simulink library "ESTS_UOD_FacOverSteer"  (R2022a)
settings: Solver=VariableStepAuto  StartTime=0.0  StopTime=10.0  RelTol=1e-3
undefined symbols (not defined in the file): ESTS_UOD_c_TiSample_s, ESTS_UOD_p_AgrVSideSlipReDifLatRefLimOS_degps, ESTS_UOD_p_TiTrans_s, ESTS_UOD_p_YawRateDifLatRefLimOS_degps
libraries: VUT_lib x3, simulink x1
settings Model: Creator=blatak  LastModifiedBy=blatak

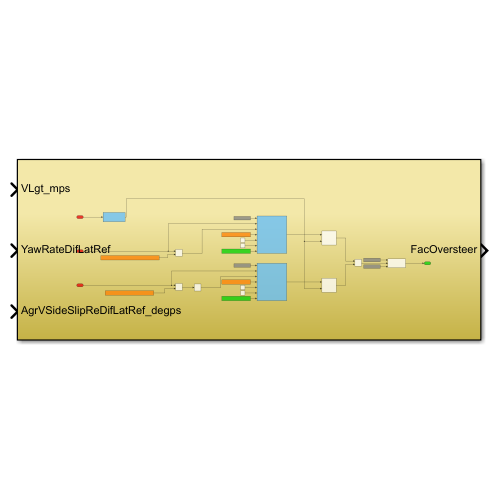
[thumbnail: Simulink's stored preview of the top-level diagram]
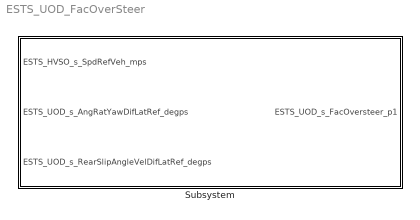
== system ESTS_UOD_FacOverSteer ==
  Subsystem : Subsystem

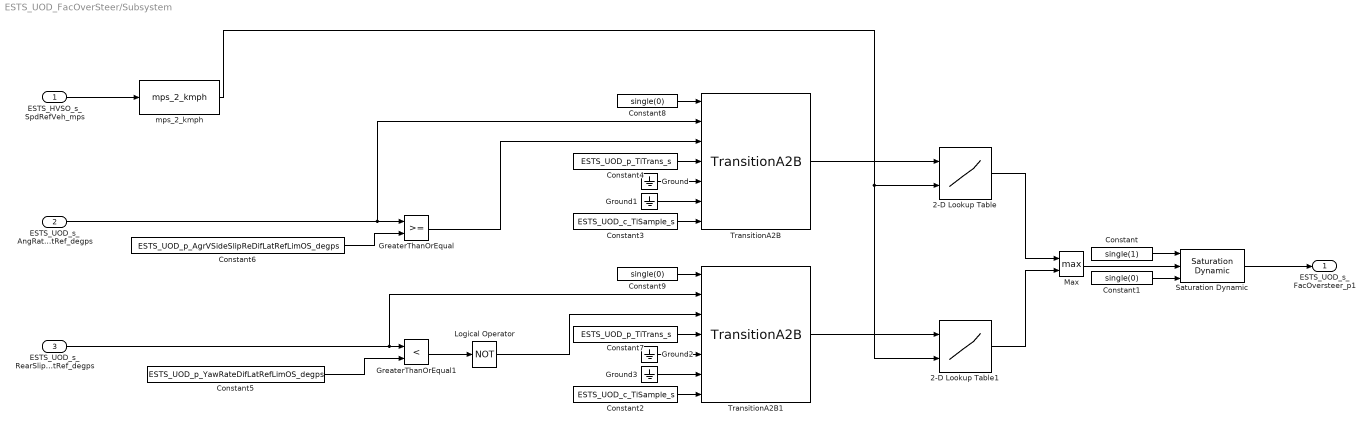
== system ESTS_UOD_FacOverSteer/Subsystem ==
  ESTS_HVSO_s_SpdRefVeh_mps : Inport
  ESTS_UOD_s_AngRatYawDifLatRef_degps : Inport  Port=2
  ESTS_UOD_s_RearSlipAngleVelDifLatRef_degps : Inport  Port=3
  2-D Lookup Table : Lookup_n-D  BreakpointsForDimension1=[1:3]  BreakpointsForDimension2=[1:3]  InternalRulePriority=Speed  RndMeth=Simplest
      settings: InputPortMap=u0,u1
  2-D Lookup Table1 : Lookup_n-D  BreakpointsForDimension1=[1:3]  BreakpointsForDimension2=[1:3]  InternalRulePriority=Speed  RndMeth=Simplest
      settings: InputPortMap=u0,u1
  Constant : Constant  Value=single(1)
  Constant1 : Constant  Value=single(0)
  Constant2 : Constant  Value=ESTS_UOD_c_TiSample_s
  Constant3 : Constant  Value=ESTS_UOD_c_TiSample_s
  Constant4 : Constant  Value=ESTS_UOD_p_TiTrans_s
  Constant5 : Constant  Value=ESTS_UOD_p_YawRateDifLatRefLimOS_degps
  Constant6 : Constant  Value=ESTS_UOD_p_AgrVSideSlipReDifLatRefLimOS_degps
  Constant7 : Constant  Value=ESTS_UOD_p_TiTrans_s
  Constant8 : Constant  Value=single(0)
  Constant9 : Constant  Value=single(0)
  GreaterThanOrEqual : RelationalOperator  OutDataTypeStr=boolean  RndMeth=Simplest  InputSameDT=off
  GreaterThanOrEqual1 : RelationalOperator  Operator=<  OutDataTypeStr=boolean  RndMeth=Simplest  InputSameDT=off
  Ground{,1..3} (4 alike) : Ground
  Logical Operator : Logic  Operator=NOT  AllPortsSameDT=off  OutDataTypeStr=boolean
  Max : MinMax  Function=max  Inputs=2
  Saturation Dynamic : simulink/Discontinuities/Saturation Dynamic  OutMin=[]  OutMax=[]  OutDataTypeStr=Inherit: Same as second input  OutDataType=fixdt(1, 16)  OutScaling=2^-10  DoSatur=off
  TransitionA2B : VUT_lib/TransitionA2B  SystemSampleTime=-1  VariantActivationTime=update diagram  Latency=0  AutoFrameSizeCalculation=off
  TransitionA2B1 : VUT_lib/TransitionA2B  SystemSampleTime=-1  VariantActivationTime=update diagram  Latency=0  AutoFrameSizeCalculation=off
  mps_2_kmph : VUT_lib/mps_2_kmph  SystemSampleTime=-1  VariantActivationTime=update diagram  Latency=0  AutoFrameSizeCalculation=off
  ESTS_UOD_s_FacOversteer_p1 : Outport
  wires:
  Ground1/1 -> TransitionA2B/6
  Constant7/1 -> TransitionA2B1/4
  Constant4/1 -> TransitionA2B/4
  mps_2_kmph/1 -> 2-D Lookup Table1/2, 2-D Lookup Table/2
  Logical Operator/1 -> TransitionA2B1/3
  Ground2/1 -> TransitionA2B1/5
  GreaterThanOrEqual1/1 -> Logical Operator/1
  ESTS_HVSO_s_SpdRefVeh_mps/1 -> mps_2_kmph/1
  GreaterThanOrEqual/1 -> TransitionA2B/3
  Constant2/1 -> TransitionA2B1/7
  Constant3/1 -> TransitionA2B/7
  Ground/1 -> TransitionA2B/5
  2-D Lookup Table/1 -> Max/1
  ESTS_UOD_s_RearSlipAngleVelDifLatRef_degps/1 -> TransitionA2B1/2, GreaterThanOrEqual1/1
  Constant9/1 -> TransitionA2B1/1
  ESTS_UOD_s_AngRatYawDifLatRef_degps/1 -> TransitionA2B/2, GreaterThanOrEqual/1
  Constant1/1 -> Saturation Dynamic/3
  TransitionA2B/1 -> 2-D Lookup Table/1
  Constant/1 -> Saturation Dynamic/1
  2-D Lookup Table1/1 -> Max/2
  Ground3/1 -> TransitionA2B1/6
  Saturation Dynamic/1 -> ESTS_UOD_s_FacOversteer_p1/1
  Max/1 -> Saturation Dynamic/2
  Constant5/1 -> GreaterThanOrEqual1/2
  Constant8/1 -> TransitionA2B/1
  Constant6/1 -> GreaterThanOrEqual/2
  TransitionA2B1/1 -> 2-D Lookup Table1/1
